simulink model "exp6_g1_p1"  (R2021b)
settings: Solver=ode45  StartTime=0.0  StopTime=10.0  RelTol=1e-3
libraries: spsMeanLib x3, spsCurrentMeasurementLib x2, spsDiodeLib x2, spsThyristorLib x2, spsVoltageMeasurementLib x2, spsACVoltageSourceLib x1, spsRMSLib x1, spsSeriesRLCBranchLib x1, spspowerguiLib x1
settings Model: Creator=marti  LastModifiedBy=marti

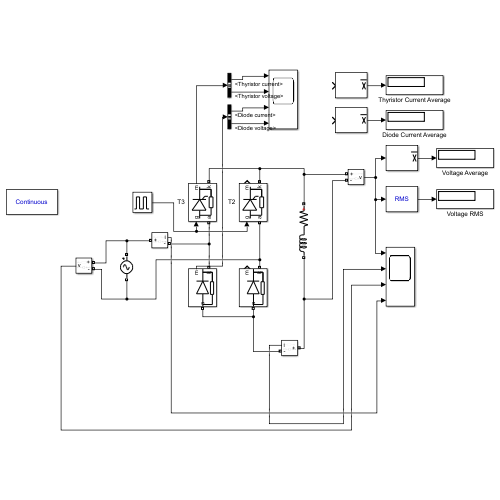
[thumbnail: Simulink's stored preview of the top-level diagram]
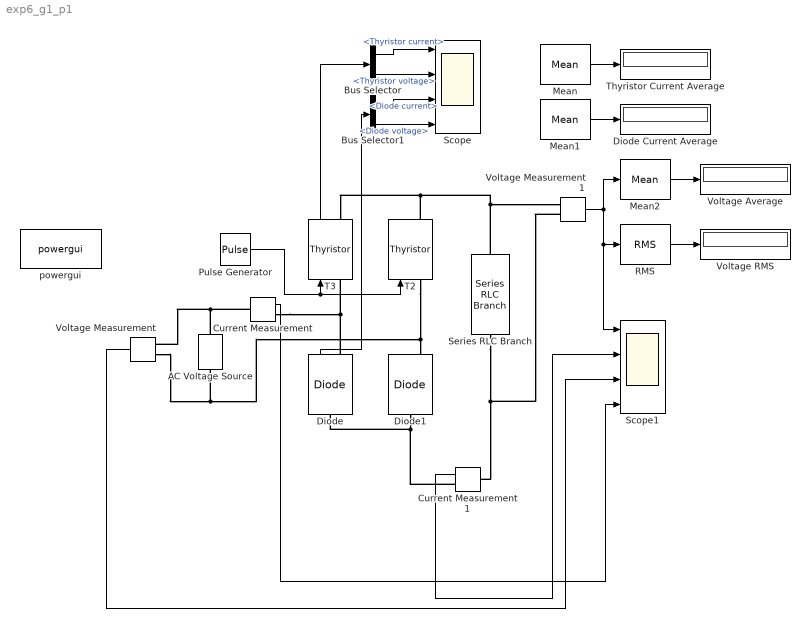
== system exp6_g1_p1 ==
  AC Voltage Source : spsACVoltageSourceLib/AC Voltage Source  Amplitude=35.35  Phase=0  Frequency=50  SampleTime=0  Measurements=None  BusType=swing  Pref=10e3  Qref=0  Qmin=-inf  Qmax=+inf
  Bus Selector : BusSelector  OutputSignals=Thyristor current,Thyristor voltage
  Bus Selector1 : BusSelector  OutputSignals=Diode current,Diode voltage
  Current Measurement : spsCurrentMeasurementLib/Current Measurement  PhasorSimulation=off  OutputType=Complex  PSBequivalent=0
  Current Measurement1 : spsCurrentMeasurementLib/Current Measurement  PhasorSimulation=off  OutputType=Complex  PSBequivalent=0
  Diode : spsDiodeLib/Diode  Ron=0.001  Lon=0  Vf=0.8  IC=0  UseSnubber=0  Rs=500  Cs=250e-9  Measurements=on
  Diode Current Average : Display
  Diode1 : spsDiodeLib/Diode  Ron=0.001  Lon=0  Vf=0.8  IC=0  UseSnubber=0  Rs=500  Cs=250e-9  Measurements=on
  Mean : spsMeanLib/Mean  Freq=60  Vinit=0  Ts=0
  Mean1 : spsMeanLib/Mean  Freq=60  Vinit=0  Ts=0
  Mean2 : spsMeanLib/Mean  Freq=60  Vinit=0  Ts=0
  Pulse Generator : DiscretePulseGenerator  PulseType=Time based  Period=0.01  PulseWidth=5  PhaseDelay=0*(0.01/180)
  RMS : spsRMSLib/RMS  TrueRMS=on  Freq=60  RMSInit=120  Ts=0
  Scope : Scope  NumInputPorts=4
  Scope1 : Scope  NumInputPorts=4
  Series RLC Branch : spsSeriesRLCBranchLib/Series RLC Branch  LConnTagsString=__new0  RConnTagsString=__new0  BranchType=RL  Resistance=12.5  Inductance=6e-3  SetiL0=off  InitialCurrent=0  Capacitance=1e-6  Setx0=off  InitialVoltage=0  Measurements=None
  T2 : spsThyristorLib/Thyristor  Ron=0.001  Lon=0  Vf=0.8  IC=0  Rs=500  Cs=250e-9  Measurements=on
  T3 : spsThyristorLib/Thyristor  Ron=0.001  Lon=0  Vf=0.8  IC=0  Rs=500  Cs=250e-9  Measurements=on
  Thyristor Current Average : Display
  Voltage Average : Display
  Voltage Measurement : spsVoltageMeasurementLib/Voltage Measurement  PhasorSimulation=off  OutputType=Complex  PSBequivalent=0
  Voltage Measurement1 : spsVoltageMeasurementLib/Voltage Measurement  PhasorSimulation=off  OutputType=Complex  PSBequivalent=0
  Voltage RMS : Display
  powergui : spspowerguiLib/powergui  Priority=1  SimulationMode=Continuous  SampleTime=50e-6  frequency=60  Iterations=50  frequencyindice=60  Pbase=100e6  ErrMax=1e-4  UnitsV=kV  UnitsW=MW  buscounter=0  FunctionMessages=off  echomessages=off  EnableUseOfTLC=off  CurrentSourceSwitches=off  DisableSnubberDevices=off  DisableRonSwitches=off  DisableVfSwitches=off  DisplayEquations=off  AutomaticDiscreteSolvers=off  SolverType=Tustin/Backward Euler (TBE)  Interpol=off  ExternalGateDelay=off  methode=off  Ts=100  x0status=blocks  SPID=on  SwTol=0  HookPort=off  NonlinearTolerance=1e-4  nMaxIteration=100  ContinueOnMaxIteration=off  RestoreLinks=warning  ResistiveCurrentMeasurement=off  Frange=[0:2:500]  Ylog=off  Xlog=on  ShowGrid=off  save=off  variable=ZData  structure=0  ZoomFFT=off  StartTime=0.0  cycles=1  DisplayStyle=1  fundamental=60  FreqAxis=off  MaxFrequency=1000  frequencyindicesteady=1  RmsSteady=1  display=off
  wires:
  Bus Selector1/1 -> Scope/3  "<Diode current>"
  Bus Selector/2 -> Scope/2  "<Thyristor voltage>"
  Bus Selector1/2 -> Scope/4  "<Diode voltage>"
  Bus Selector/1 -> Scope/1  "<Thyristor current>"
  Pulse Generator/1 -> T2/1, T3/1
  T3/1 -> Bus Selector/1
  Diode/1 -> Bus Selector1/1
  Mean/1 -> Thyristor Current Average/1
  Mean1/1 -> Diode Current Average/1
  Mean2/1 -> Voltage Average/1
  RMS/1 -> Voltage RMS/1
  Voltage Measurement1/1 -> Mean2/1, RMS/1, Scope1/1
  Current Measurement1/1 -> Scope1/2
  Voltage Measurement/1 -> Scope1/3
  Current Measurement/1 -> Scope1/4
  connections:
  Series RLC Branch/RConn1 -- Voltage Measurement1/LConn2 -- Current Measurement1/LConn1
  Diode1/LConn1 -- Current Measurement1/RConn1 -- Diode/LConn1
  T2/LConn1 -- AC Voltage Source/LConn1 -- Voltage Measurement/LConn2 -- Diode1/RConn1
  Diode/RConn1 -- T3/LConn1 -- Current Measurement/RConn1
  Current Measurement/LConn1 -- Voltage Measurement/LConn1 -- AC Voltage Source/RConn1
  Series RLC Branch/LConn1 -- T3/RConn1 -- T2/RConn1 -- Voltage Measurement1/LConn1
